simulink model "Indicators"  (R2023b)
settings: Solver=FixedStepAuto  StartTime=0.0  StopTime=inf  FixedStep=1  RelTol=1e-3  EnableMultiTasking=on
libraries: arduinolib x5, dspswit3 x3
settings Model: ExtModeTrigDuration=2  Creator=MOHAMED  LastModifiedBy=MOHAMED
settings OptimizationCC: EnhancedBackFolding=on  PassReuseOutputArgsAs=Individual arguments  ZeroExternalMemoryAtStartup=off  ZeroInternalMemoryAtStartup=off  MaxStackSize=64  OptimizeBlockOrder=speed  DifferentSizesBufferReuse=on  OptimizationCustomize=off  EfficientTunableParamExpr=on
settings DebuggingCC: ParameterTunabilityLossMsg=error
settings HardwareCC: ProdBitPerInt=16  ProdBitPerPointer=16  ProdBitPerSizeT=16  ProdBitPerPtrDiffT=16  ProdLargestAtomicFloat=None  ProdWordSize=8  ProdHWDeviceType=Atmel->AVR
settings SFSimCC: MATLABDynamicMemAlloc=off
settings RTWCC: Description=Embedded Coder  SystemTargetFile=ert.tlc  HardwareBoard=Arduino Uno  TemplateMakefile=ert_default_tmf  Toolchain=Arduino AVR  BuildConfiguration=Faster Runs
settings CodeAppCC: ForceParamTrailComments=on  IgnoreCustomStorageClasses=off  OperatorAnnotations=on  SimulinkDataObjDesc=on  SFDataObjDesc=on  InsertBlockDesc=on
settings ERTTargetCC: SupportContinuousTime=on  SupportVariableSizeSignals=on  ExtModeTransport=3  ExtModeStaticAlloc=on  ExtModeAutomaticAllocSize=off  ExtModeStaticAllocSize=250  ExtModeMexFile=ext_xcp  ExtModeIntrfLevel=Level2 - Open

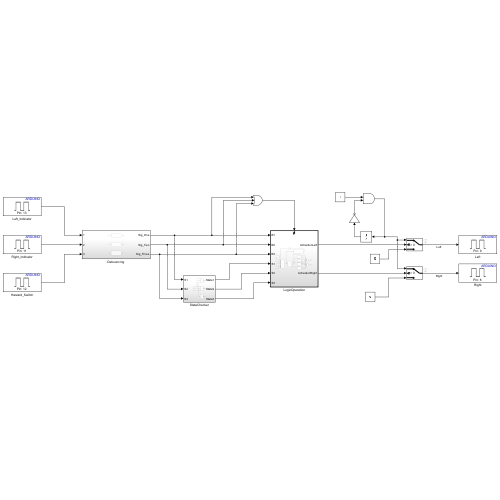
[thumbnail: Simulink's stored preview of the top-level diagram]
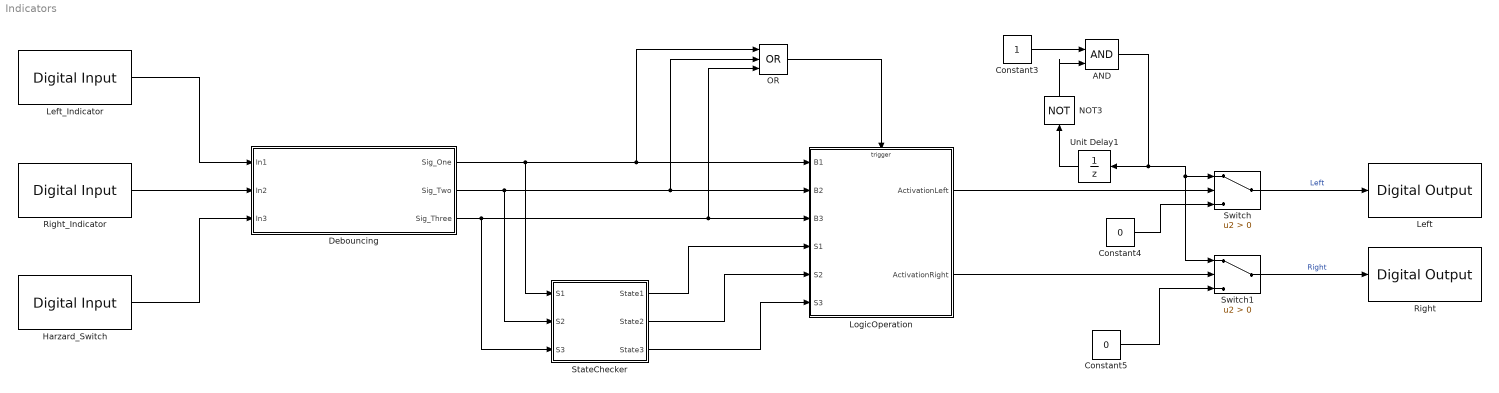
== system Indicators ==
  AND : Logic  IconShape=distinctive  AllPortsSameDT=off  OutDataTypeStr=boolean
  Constant3 : Constant
  Constant4 : Constant  Value=0
  Constant5 : Constant  Value=0
  "Debouncing " : Subsystem
  Harzard_Switch : arduinolib/Digital Input  pinNumber=12  mode=Input Pullup  Direction=input  SampleTime=1  blockPlatform=arduino
  Left : arduinolib/Digital Output  pinNumber=9  Direction=output  blockPlatform=arduino
  Left_Indicator : arduinolib/Digital Input  pinNumber=13  mode=Input Pullup  Direction=input  SampleTime=1  blockPlatform=arduino
  LogicOperation : Subsystem
  NOT3 : Logic  Operator=NOT  IconShape=distinctive  AllPortsSameDT=off  OutDataTypeStr=boolean
  OR : Logic  Operator=OR  Inputs=3  IconShape=distinctive  AllPortsSameDT=off  OutDataTypeStr=boolean
  Right : arduinolib/Digital Output  pinNumber=8  Direction=output  blockPlatform=arduino
  Right_Indicator : arduinolib/Digital Input  pinNumber=11  mode=Input Pullup  Direction=input  SampleTime=1  blockPlatform=arduino
  StateChecker : Subsystem
  Switch : Switch  Criteria=u2 > Threshold  SaturateOnIntegerOverflow=off  InputSameDT=off
  Switch1 : Switch  Criteria=u2 > Threshold  SaturateOnIntegerOverflow=off  InputSameDT=off
  Unit Delay1 : UnitDelay  InitialCondition=1  SampleTime=-1  HasFrameUpgradeWarning=on
  wires:
  "Debouncing "/1(Sig_One) -> StateChecker/1(S1), OR/1, LogicOperation/1(B1)
  "Debouncing "/2(Sig_Two) -> StateChecker/2(S2), OR/2, LogicOperation/2(B2)
  "Debouncing "/3(Sig_Three) -> StateChecker/3(S3), OR/3, LogicOperation/3(B3)
  StateChecker/1(State1) -> LogicOperation/4(S1)
  StateChecker/2(State2) -> LogicOperation/5(S2)
  StateChecker/3(State3) -> LogicOperation/6(S3)
  OR/1 -> LogicOperation/Trigger
  Constant5/1 -> Switch1/3
  AND/1 -> Switch1/1, Switch/1, Unit Delay1/1
  Switch/1 -> Left/1  "Left"
  Constant4/1 -> Switch/3
  NOT3/1 -> AND/2
  Switch1/1 -> Right/1  "Right"
  Unit Delay1/1 -> NOT3/1
  Constant3/1 -> AND/1
  LogicOperation/1(ActivationLeft) -> Switch/2
  LogicOperation/2(ActivationRight) -> Switch1/2
  Left_Indicator/1 -> "Debouncing "/1(In1)
  Right_Indicator/1 -> "Debouncing "/2(In2)
  Harzard_Switch/1 -> "Debouncing "/3(In3)

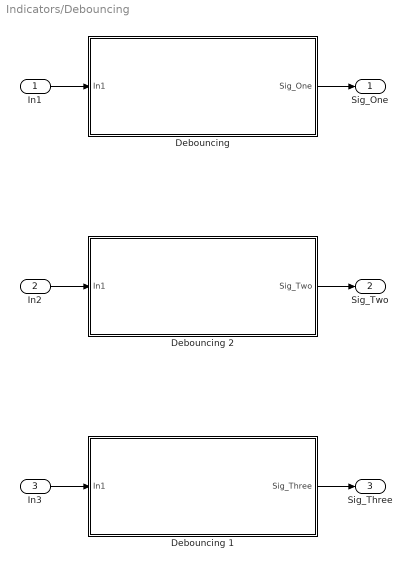
== system Indicators/Debouncing  ==
  In1 : Inport
  In2 : Inport  Port=2
  In3 : Inport  Port=3
  "Debouncing " : Subsystem
  Debouncing 1 : Subsystem
  Debouncing 2 : Subsystem
  Sig_One : Outport
  Sig_Two : Outport  Port=2
  Sig_Three : Outport  Port=3
  wires:
  "Debouncing "/1(Sig_One) -> Sig_One/1
  Debouncing 1/1(Sig_Three) -> Sig_Three/1
  Debouncing 2/1(Sig_Two) -> Sig_Two/1
  In3/1 -> Debouncing 1/1(In1)
  In2/1 -> Debouncing 2/1(In1)
  In1/1 -> "Debouncing "/1(In1)

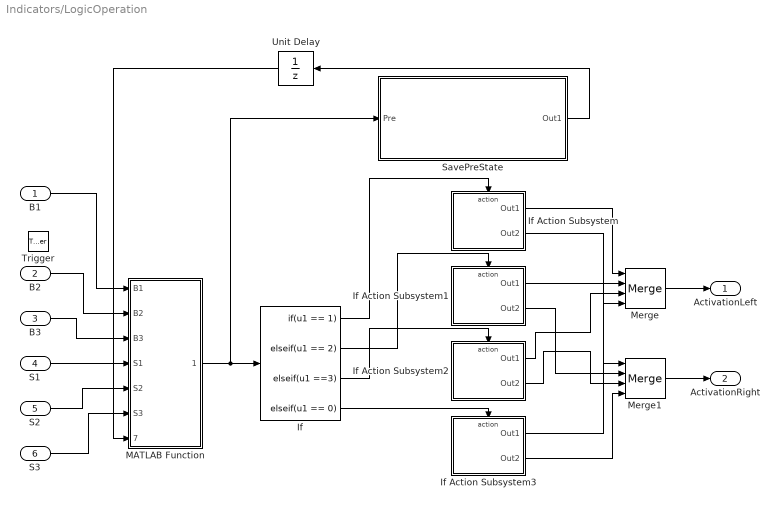
== system Indicators/LogicOperation ==
  B1 : Inport
  B2 : Inport  Port=2
  B3 : Inport  Port=3
  S1 : Inport  Port=4
  S2 : Inport  Port=5
  S3 : Inport  Port=6
  Trigger : TriggerPort  VariantControl=(inherit)  PortDimensions=1
  If : If  IfExpression=u1 == 1  ElseIfExpressions=u1 == 2 , u1 ==3, u1 == 0  ShowElse=off
  If Action Subsystem : Subsystem  TreatAsAtomicUnit=on
  If Action Subsystem1 : Subsystem  TreatAsAtomicUnit=on
  If Action Subsystem2 : Subsystem  TreatAsAtomicUnit=on
  If Action Subsystem3 : Subsystem  TreatAsAtomicUnit=on
  MATLAB Function : MATLAB Function  TreatAsAtomicUnit=on
  Merge : Merge  Inputs=4
  Merge1 : Merge  Inputs=4
  SavePreState : Subsystem
  Unit Delay : UnitDelay  SampleTime=-1  HasFrameUpgradeWarning=on
  ActivationLeft : Outport
  ActivationRight : Outport  Port=2
  wires:
  If Action Subsystem/1(Out1) -> Merge/1
  S3/1 -> MATLAB Function/6(S3)
  If Action Subsystem2/2(Out2) -> Merge1/3
  S2/1 -> MATLAB Function/5(S2)
  If Action Subsystem/2(Out2) -> Merge1/1
  S1/1 -> MATLAB Function/4(S1)
  If/4 -> If Action Subsystem3/Action
  B3/1 -> MATLAB Function/3(B3)
  If Action Subsystem1/2(Out2) -> Merge1/2
  If/3 -> If Action Subsystem2/Action
  B2/1 -> MATLAB Function/2(B2)
  If/2 -> If Action Subsystem1/Action
  B1/1 -> MATLAB Function/1(B1)
  If Action Subsystem3/2(Out2) -> Merge1/4
  MATLAB Function/1(Activation) -> SavePreState/1(Pre), If/1
  Unit Delay/1 -> MATLAB Function/7(PreState)
  If/1 -> If Action Subsystem/Action
  SavePreState/1(Out1) -> Unit Delay/1
  If Action Subsystem1/1(Out1) -> Merge/2
  If Action Subsystem2/1(Out1) -> Merge/3
  If Action Subsystem3/1(Out1) -> Merge/4
  Merge/1 -> ActivationLeft/1
  Merge1/1 -> ActivationRight/1

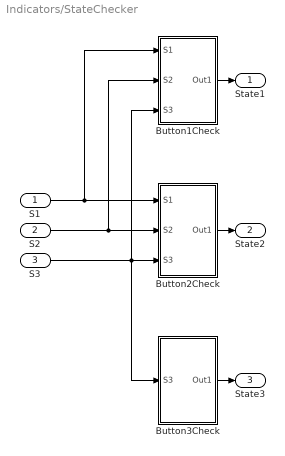
== system Indicators/StateChecker ==
  S1 : Inport
  S2 : Inport  Port=2
  S3 : Inport  Port=3
  Button1Check : Subsystem
  Button2Check : Subsystem
  Button3Check : Subsystem
  State1 : Outport
  State2 : Outport  Port=2
  State3 : Outport  Port=3
  wires:
  S1/1 -> Button2Check/1(S1), Button1Check/1(S1)
  S2/1 -> Button1Check/2(S2), Button2Check/2(S2)
  Button1Check/1(Out1) -> State1/1
  S3/1 -> Button1Check/3(S3), Button2Check/3(S3), Button3Check/1(S3)
  Button2Check/1(Out1) -> State2/1
  Button3Check/1(Out1) -> State3/1

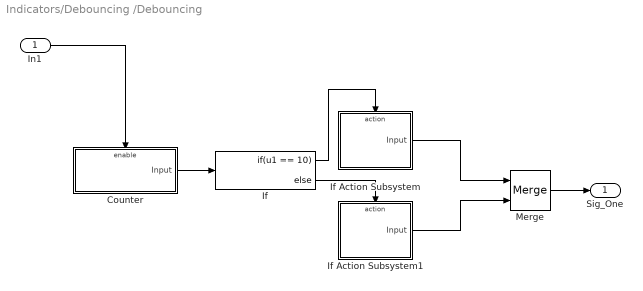
== system Indicators/Debouncing /Debouncing  ==
  In1 : Inport
  Counter : Subsystem  TreatAsAtomicUnit=on
  If : If  IfExpression=u1 == 10
  If Action Subsystem : Subsystem  TreatAsAtomicUnit=on
  If Action Subsystem1 : Subsystem  TreatAsAtomicUnit=on
  Merge : Merge
  Sig_One : Outport
  wires:
  Counter/1(Input) -> If/1
  In1/1 -> Counter/Enable
  If/1 -> If Action Subsystem/Action
  If/2 -> If Action Subsystem1/Action
  Merge/1 -> Sig_One/1
  If Action Subsystem/1(Input) -> Merge/1
  If Action Subsystem1/1(Input) -> Merge/2

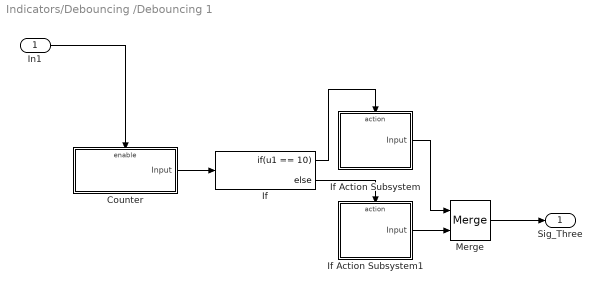
== system Indicators/Debouncing /Debouncing 1 ==
  In1 : Inport
  Counter : Subsystem  TreatAsAtomicUnit=on
  If : If  IfExpression=u1 == 10
  If Action Subsystem : Subsystem  TreatAsAtomicUnit=on
  If Action Subsystem1 : Subsystem  TreatAsAtomicUnit=on
  Merge : Merge
  Sig_Three : Outport
  wires:
  If/2 -> If Action Subsystem1/Action
  If/1 -> If Action Subsystem/Action
  In1/1 -> Counter/Enable
  If Action Subsystem1/1(Input) -> Merge/2
  Merge/1 -> Sig_Three/1
  Counter/1(Input) -> If/1
  If Action Subsystem/1(Input) -> Merge/1

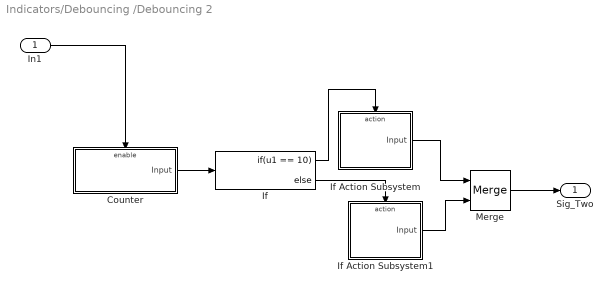
== system Indicators/Debouncing /Debouncing 2 ==
  In1 : Inport
  Counter : Subsystem  TreatAsAtomicUnit=on
  If : If  IfExpression=u1 == 10
  If Action Subsystem : Subsystem  TreatAsAtomicUnit=on
  If Action Subsystem1 : Subsystem  TreatAsAtomicUnit=on
  Merge : Merge
  Sig_Two : Outport
  wires:
  Counter/1(Input) -> If/1
  In1/1 -> Counter/Enable
  If/1 -> If Action Subsystem/Action
  If/2 -> If Action Subsystem1/Action
  If Action Subsystem/1(Input) -> Merge/1
  If Action Subsystem1/1(Input) -> Merge/2
  Merge/1 -> Sig_Two/1

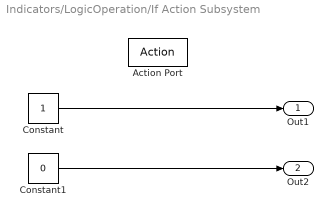
== system Indicators/LogicOperation/If Action Subsystem ==
  Action Port : ActionPort  ActionPortLabel=if(u1 == 1)
  Constant : Constant
  Constant1 : Constant  Value=0
  Out1 : Outport
  Out2 : Outport  Port=2
  wires:
  Constant/1 -> Out1/1
  Constant1/1 -> Out2/1

== system Indicators/LogicOperation/If Action Subsystem1 ==
  Action Port : ActionPort  ActionPortLabel=elseif(u1 == 2 )
  Constant : Constant  Value=0
  Constant1 : Constant
  Out1 : Outport
  Out2 : Outport  Port=2
  wires:
  Constant1/1 -> Out2/1
  Constant/1 -> Out1/1

== system Indicators/LogicOperation/If Action Subsystem2 ==
  Action Port : ActionPort  ActionPortLabel=elseif( u1 ==3)
  Constant : Constant
  Constant1 : Constant
  Out1 : Outport
  Out2 : Outport  Port=2
  wires:
  Constant/1 -> Out1/1
  Constant1/1 -> Out2/1

== system Indicators/LogicOperation/If Action Subsystem3 ==
  Action Port : ActionPort  ActionPortLabel=elseif( u1 == 0)
  Constant : Constant  Value=0
  Constant1 : Constant  Value=0
  Out1 : Outport
  Out2 : Outport  Port=2
  wires:
  Constant1/1 -> Out2/1
  Constant/1 -> Out1/1

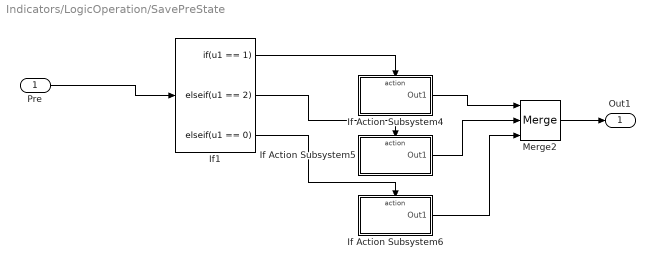
== system Indicators/LogicOperation/SavePreState ==
  Pre : Inport
  If Action Subsystem4 : Subsystem  TreatAsAtomicUnit=on
  If Action Subsystem5 : Subsystem  TreatAsAtomicUnit=on
  If Action Subsystem6 : Subsystem  TreatAsAtomicUnit=on
  If1 : If  IfExpression=u1 == 1  ElseIfExpressions=u1 == 2 , u1 == 0  ShowElse=off
  Merge2 : Merge  Inputs=3
  Out1 : Outport
  wires:
  If Action Subsystem4/1(Out1) -> Merge2/1
  If Action Subsystem6/1(Out1) -> Merge2/3
  If1/3 -> If Action Subsystem6/Action
  If1/1 -> If Action Subsystem4/Action
  Merge2/1 -> Out1/1
  If Action Subsystem5/1(Out1) -> Merge2/2
  If1/2 -> If Action Subsystem5/Action
  Pre/1 -> If1/1

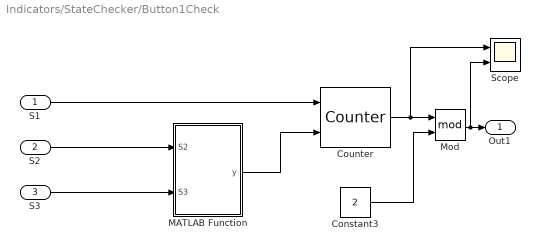
== system Indicators/StateChecker/Button1Check ==
  S1 : Inport
  S2 : Inport  Port=2
  S3 : Inport  Port=3
  Constant3 : Constant  Value=2
  Counter : dspswit3/Counter  Direction=Up  CountEvent=Rising edge  CounterSize=User defined  MaxCount=255  InitialCount=0  Output=Count  HitValue=32  ResetInput=on  SamplesPerFrame=1  Ts=1  CntDtype=double  HitDtype=Logical
  MATLAB Function : MATLAB Function  TreatAsAtomicUnit=on
  Mod : Math  Operator=mod
  Scope : Scope  NumInputPorts=2
  Out1 : Outport
  wires:
  MATLAB Function/1(y) -> Counter/2
  Constant3/1 -> Mod/2
  Counter/1 -> Scope/1, Mod/1
  S3/1 -> MATLAB Function/2(S3)
  Mod/1 -> Scope/2, Out1/1
  S1/1 -> Counter/1
  S2/1 -> MATLAB Function/1(S2)

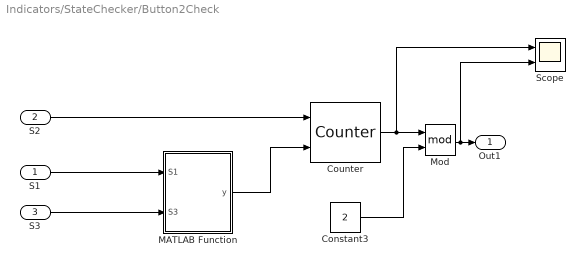
== system Indicators/StateChecker/Button2Check ==
  S1 : Inport
  S2 : Inport  Port=2
  S3 : Inport  Port=3
  Constant3 : Constant  Value=2
  Counter : dspswit3/Counter  Direction=Up  CountEvent=Rising edge  CounterSize=User defined  MaxCount=255  InitialCount=0  Output=Count  HitValue=32  ResetInput=on  SamplesPerFrame=1  Ts=1  CntDtype=double  HitDtype=Logical
  MATLAB Function : MATLAB Function  TreatAsAtomicUnit=on
  Mod : Math  Operator=mod
  Scope : Scope  NumInputPorts=2
  Out1 : Outport
  wires:
  Mod/1 -> Scope/2, Out1/1
  S3/1 -> MATLAB Function/2(S3)
  Counter/1 -> Scope/1, Mod/1
  Constant3/1 -> Mod/2
  MATLAB Function/1(y) -> Counter/2
  S2/1 -> Counter/1
  S1/1 -> MATLAB Function/1(S1)

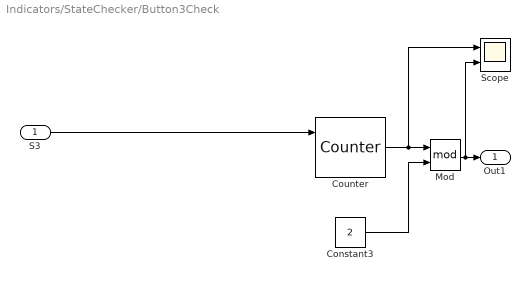
== system Indicators/StateChecker/Button3Check ==
  S3 : Inport
  Constant3 : Constant  Value=2
  Counter : dspswit3/Counter  Direction=Up  CountEvent=Rising edge  CounterSize=User defined  MaxCount=255  InitialCount=0  Output=Count  HitValue=32  ResetInput=on  SamplesPerFrame=1  Ts=1  CntDtype=double  HitDtype=Logical
  Mod : Math  Operator=mod
  Scope : Scope  NumInputPorts=2
  Out1 : Outport
  wires:
  Constant3/1 -> Mod/2
  Counter/1 -> Scope/1, Mod/1
  Mod/1 -> Scope/2, Out1/1
  S3/1 -> Counter/1

== system Indicators/Debouncing /Debouncing /Counter ==
  Enable : EnablePort  StatesWhenEnabling=reset
  Constant : Constant
  Sum : Sum  Inputs=|++
  Unit Delay : UnitDelay  SampleTime=-1  HasFrameUpgradeWarning=on
  Input : Outport
  wires:
  Sum/1 -> Unit Delay/1, Input/1
  Constant/1 -> Sum/1
  Unit Delay/1 -> Sum/2

== system Indicators/Debouncing /Debouncing /If Action Subsystem ==
  Action Port : ActionPort  ActionPortLabel=if(u1 == 10)
  Constant : Constant
  Input : Outport
  wires:
  Constant/1 -> Input/1

== system Indicators/Debouncing /Debouncing /If Action Subsystem1 ==
  Action Port : ActionPort  InitializeStates=reset  ActionPortLabel=else
  Constant : Constant  Value=0
  Input : Outport
  wires:
  Constant/1 -> Input/1

== system Indicators/Debouncing /Debouncing 1/Counter ==
  Enable : EnablePort  StatesWhenEnabling=reset
  Constant : Constant
  Sum : Sum  Inputs=|++
  Unit Delay : UnitDelay  SampleTime=-1  HasFrameUpgradeWarning=on
  Input : Outport
  wires:
  Unit Delay/1 -> Sum/2
  Constant/1 -> Sum/1
  Sum/1 -> Input/1, Unit Delay/1

== system Indicators/Debouncing /Debouncing 1/If Action Subsystem ==
  Action Port : ActionPort  ActionPortLabel=if(u1 == 10)
  Constant : Constant
  Input : Outport
  wires:
  Constant/1 -> Input/1

== system Indicators/Debouncing /Debouncing 1/If Action Subsystem1 ==
  Action Port : ActionPort  ActionPortLabel=else
  Constant : Constant  Value=0
  Input : Outport
  wires:
  Constant/1 -> Input/1

== system Indicators/Debouncing /Debouncing 2/Counter ==
  Enable : EnablePort  StatesWhenEnabling=reset
  Constant : Constant
  Sum : Sum  Inputs=|++
  Unit Delay : UnitDelay  SampleTime=-1  HasFrameUpgradeWarning=on
  Input : Outport
  wires:
  Sum/1 -> Unit Delay/1, Input/1
  Constant/1 -> Sum/1
  Unit Delay/1 -> Sum/2

== system Indicators/Debouncing /Debouncing 2/If Action Subsystem ==
  Action Port : ActionPort  ActionPortLabel=if(u1 == 10)
  Constant : Constant
  Input : Outport
  wires:
  Constant/1 -> Input/1

== system Indicators/Debouncing /Debouncing 2/If Action Subsystem1 ==
  Action Port : ActionPort  ActionPortLabel=else
  Constant : Constant  Value=0
  Input : Outport
  wires:
  Constant/1 -> Input/1

== system Indicators/LogicOperation/SavePreState/If Action Subsystem4 ==
  Action Port : ActionPort  ActionPortLabel=if(u1 == 1)
  Constant : Constant
  Out1 : Outport
  wires:
  Constant/1 -> Out1/1

== system Indicators/LogicOperation/SavePreState/If Action Subsystem5 ==
  Action Port : ActionPort  ActionPortLabel=elseif(u1 == 2 )
  Constant : Constant  Value=2
  Out1 : Outport
  wires:
  Constant/1 -> Out1/1

== system Indicators/LogicOperation/SavePreState/If Action Subsystem6 ==
  Action Port : ActionPort  ActionPortLabel=elseif( u1 == 0)
  Constant : Constant  Value=0
  Out1 : Outport
  wires:
  Constant/1 -> Out1/1

== matlab function Indicators/StateChecker/Button2Check/MATLAB Function ==
  data: S1 input; y output; S3 input
function y = fcn(S1, S3)
y = 0;
if (S1 == 1 || S3 == 1)
    y = 1;
end

== matlab function Indicators/StateChecker/Button1Check/MATLAB Function ==
  data: S2 input; y output; S3 input
function y = fcn(S2, S3)
y = 0;
if (S2 == 1 || S3 == 1)
    y = 1;
end

== matlab function Indicators/LogicOperation/MATLAB Function ==
  data: B1 input; Activation output; B2 input; B3 input; S1 input; S2 input; S3 input; PreState input
function Activation = fcn(B1, B2, B3, S1, S2, S3, PreState)

Activation = 0;

if (S3 == 1)
    Activation = 3;
elseif (B1 == 1 && B2 == 0 && B3 == 0 && S1 == 1)
    Activation = 1;
elseif (B1 == 1 && B2 == 0 && B3 == 0 && S1 == 0) || (B1 == 0 && B2 == 1 && B3 == 0 && S2 == 0)
    Activation = 0;
elseif (B1 == 0 && B2 == 1 && B3 == 0 && S2 == 1)
    Activation = 2;
elseif (B1 == 0 && B2 == 0 && S3 == 1)
    Activation = 3;
elseif (B1 == 0 && B2 == 0 && S3 == 0)
    Activation = PreState;
end

if (PreState == 0 && S3 == 0 && B1 == 0 && B2 == 0)
    Activation = 0;
elseif (PreState == 1 && S3 == 0 && S1 == 0 && B1 == 0 && B2 == 0)
    Activation = 1;
elseif (PreState == 2 && S3 == 0 && S2 == 0 && B1 == 0 && B2 == 0)
    Activation = 2;
end
